simulink model "trefas"  (R2022b)
settings: Solver=VariableStepAuto  StartTime=0.0  StopTime=0.1  RelTol=1e-7
model workspace (MAT data in the model file):
  L = Simulink.Parameter
  L.Value = 0.095
  L.DataType = 'auto'
  L.Complexity = 'real'
  L.Dimensions = [1 1]
  R = 40
  a = 220
  freq = 314.16
values from neighbouring files (symbols this model uses):
  L = 0.095    [lab1.m]
settings Model: Creator=axelfroborg  LastModifiedBy=emill
settings SolverCC: AlgebraicLoopSolver=TrustRegion
settings DebuggingCC: UnconnectedInputMsg=warning  UnconnectedOutputMsg=warning  UnconnectedLineMsg=warning  SFMachineParentedDataDiag=warning
settings ModelReferenceCC: EnableRefExpFcnMdlSchedulingChecks=on
settings RTWCC: DLArmComputeVersion=19.05

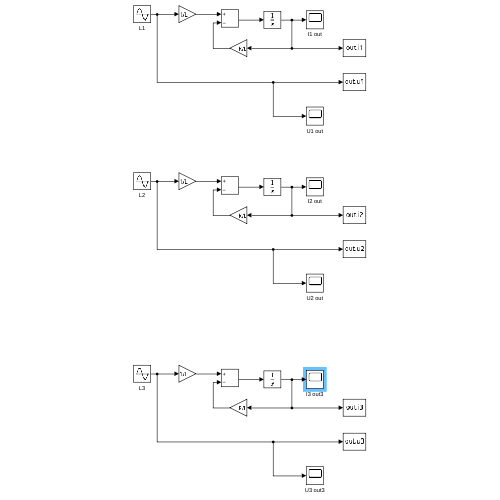
[thumbnail: Simulink's stored preview of the top-level diagram]
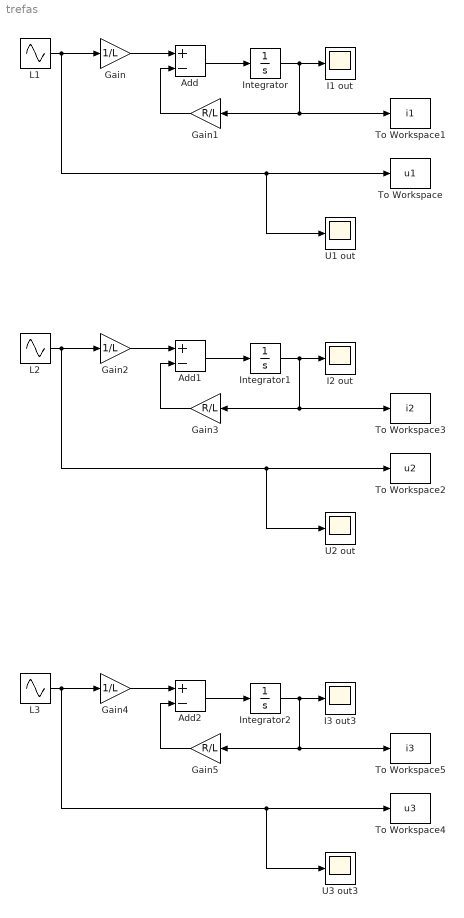
== system trefas ==
  Add : Sum  Inputs=+-
  Add1 : Sum  Inputs=+-
  Add2 : Sum  Inputs=+-
  Gain : Gain  Gain=1/L
  Gain1 : Gain  Gain=R/L
  Gain2 : Gain  Gain=1/L
  Gain3 : Gain  Gain=R/L
  Gain4 : Gain  Gain=1/L
  Gain5 : Gain  Gain=R/L
  I1 out : Scope
  I2 out : Scope
  I3 out3 : Scope
  Integrator : Integrator
  Integrator1 : Integrator
  Integrator2 : Integrator
  L1 : Sin  Amplitude=220  Frequency=freq  SampleTime=0
  L2 : Sin  Amplitude=220  Frequency=freq  Phase=2/3*pi  SampleTime=0
  L3 : Sin  Amplitude=220  Frequency=freq  Phase=4/3*pi  SampleTime=0
  To Workspace : ToWorkspace  VariableName=u1  SampleTime=-1
  To Workspace1 : ToWorkspace  VariableName=i1  SampleTime=-1
  To Workspace2 : ToWorkspace  VariableName=u2  SampleTime=-1
  To Workspace3 : ToWorkspace  VariableName=i2  SampleTime=-1
  To Workspace4 : ToWorkspace  VariableName=u3  SampleTime=-1
  To Workspace5 : ToWorkspace  VariableName=i3  SampleTime=-1
  U1 out : Scope
  U2 out : Scope
  U3 out3 : Scope
  wires:
  Integrator/1 -> Gain1/1, To Workspace1/1, I1 out/1
  Gain1/1 -> Add/2
  L1/1 -> Gain/1, U1 out/1, To Workspace/1
  Gain/1 -> Add/1
  Add/1 -> Integrator/1
  Add1/1 -> Integrator1/1
  Integrator1/1 -> Gain3/1, To Workspace3/1, I2 out/1
  Gain3/1 -> Add1/2
  L2/1 -> Gain2/1, U2 out/1, To Workspace2/1
  Gain2/1 -> Add1/1
  L3/1 -> Gain4/1, U3 out3/1, To Workspace4/1
  Integrator2/1 -> Gain5/1, To Workspace5/1, I3 out3/1
  Gain4/1 -> Add2/1
  Add2/1 -> Integrator2/1
  Gain5/1 -> Add2/2
